simulink model "sha2_net_design"  (R2018b)
settings: Solver=VariableStepAuto  StartTime=0.0  StopTime=10.0  RelTol=1e-3
settings Model: Creator=Mihail  LastModifiedBy=Mihail

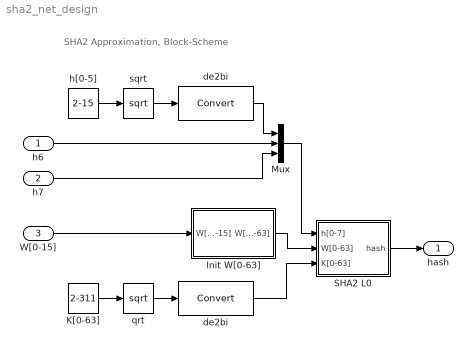
== system sha2_net_design ==
  note: SHA2 Approximation, Block-Scheme
  h6 : Inport
  h7 : Inport  Port=2
  W[0-15] : Inport  Port=3
  Init W[0-63] : Subsystem
  K[0-63] : Constant  Value=2-311
  Mux : Mux  Inputs=3
  SHA2 L0 : Subsystem
  de2bi : DataTypeConversion
  "de2bi " : DataTypeConversion
  h[0-5] : Constant  Value=2-15
  qrt : Sqrt  SaturateOnIntegerOverflow=on
  sqrt : Sqrt  SaturateOnIntegerOverflow=on
  hash : Outport
  wires:
  h[0-5]/1 -> sqrt/1
  K[0-63]/1 -> qrt/1
  sqrt/1 -> de2bi/1
  de2bi/1 -> Mux/1
  h6/1 -> Mux/2
  h7/1 -> Mux/3
  qrt/1 -> "de2bi "/1
  Init W[0-63]/1("W[0-63] ") -> SHA2 L0/2(W[0-63])
  Mux/1 -> SHA2 L0/1(h[0-7])
  "de2bi "/1 -> SHA2 L0/3(K[0-63])
  W[0-15]/1 -> Init W[0-63]/1(W[0-15])
  SHA2 L0/1(hash) -> hash/1

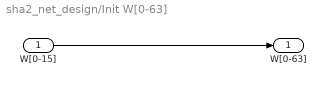
== system sha2_net_design/Init W[0-63] ==
  W[0-15] : Inport
  "W[0-63] " : Outport
  wires:
  W[0-15]/1 -> "W[0-63] "/1

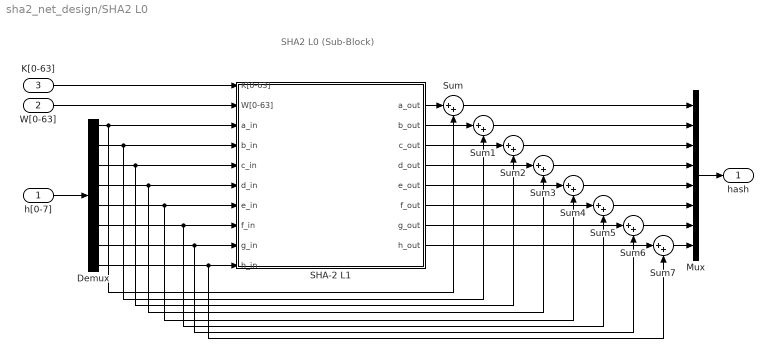
== system sha2_net_design/SHA2 L0 ==
  note: SHA2 L0 (Sub-Block)
  h[0-7] : Inport
  W[0-63] : Inport  Port=2
  K[0-63] : Inport  Port=3
  Demux : Demux  Outputs=8
  Mux : Mux  Inputs=8
  SHA-2 L1 : Subsystem
  Sum{,1..7} (8 alike) : Sum  Inputs=|++
  hash : Outport
  wires:
  SHA-2 L1/1(a_out) -> Sum/1
  SHA-2 L1/2(b_out) -> Sum1/1
  Sum/1 -> Mux/1
  Sum1/1 -> Mux/2
  Sum2/1 -> Mux/3
  SHA-2 L1/3(c_out) -> Sum2/1
  SHA-2 L1/4(d_out) -> Sum3/1
  Sum3/1 -> Mux/4
  SHA-2 L1/5(e_out) -> Sum4/1
  Sum4/1 -> Mux/5
  Mux/1 -> hash/1
  SHA-2 L1/6(f_out) -> Sum5/1
  Sum6/1 -> Mux/7
  Sum5/1 -> Mux/6
  Sum7/1 -> Mux/8
  SHA-2 L1/7(g_out) -> Sum6/1
  SHA-2 L1/8(h_out) -> Sum7/1
  W[0-63]/1 -> SHA-2 L1/2(W[0-63])
  K[0-63]/1 -> SHA-2 L1/1(K[0-63])
  h[0-7]/1 -> Demux/1
  Demux/1 -> Sum/2, SHA-2 L1/3(a_in)
  Demux/2 -> Sum1/2, SHA-2 L1/4(b_in)
  Demux/3 -> Sum2/2, SHA-2 L1/5(c_in)
  Demux/4 -> Sum3/2, SHA-2 L1/6(d_in)
  Demux/5 -> Sum4/2, SHA-2 L1/7(e_in)
  Demux/6 -> Sum5/2, SHA-2 L1/8(f_in)
  Demux/7 -> Sum6/2, SHA-2 L1/9(g_in)
  Demux/8 -> Sum7/2, SHA-2 L1/10(h_in)

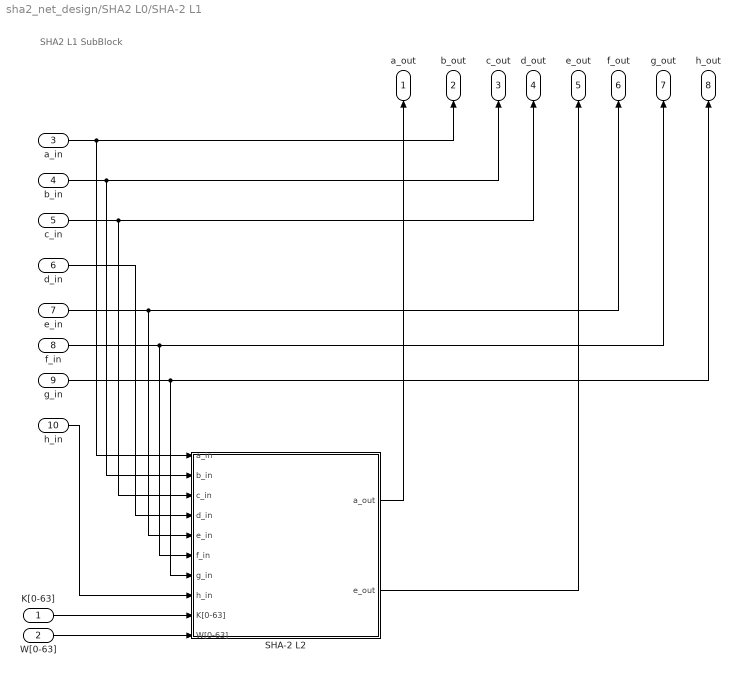
== system sha2_net_design/SHA2 L0/SHA-2 L1 ==
  note: SHA2 L1 SubBlock
  K[0-63] : Inport
  W[0-63] : Inport  Port=2
  a_in : Inport  Port=3
  b_in : Inport  Port=4
  c_in : Inport  Port=5
  d_in : Inport  Port=6
  e_in : Inport  Port=7
  f_in : Inport  Port=8
  g_in : Inport  Port=9
  h_in : Inport  Port=10
  SHA-2 L2 : Subsystem
  a_out : Outport
  b_out : Outport  Port=2
  c_out : Outport  Port=3
  d_out : Outport  Port=4
  e_out : Outport  Port=5
  f_out : Outport  Port=6
  g_out : Outport  Port=7
  h_out : Outport  Port=8
  wires:
  g_in/1 -> SHA-2 L2/7(g_in), h_out/1
  f_in/1 -> SHA-2 L2/6(f_in), g_out/1
  e_in/1 -> SHA-2 L2/5(e_in), f_out/1
  c_in/1 -> SHA-2 L2/3(c_in), d_out/1
  b_in/1 -> SHA-2 L2/2(b_in), c_out/1
  a_in/1 -> SHA-2 L2/1(a_in), b_out/1
  SHA-2 L2/1(a_out) -> a_out/1
  SHA-2 L2/2(e_out) -> e_out/1
  d_in/1 -> SHA-2 L2/4(d_in)
  h_in/1 -> SHA-2 L2/8(h_in)
  K[0-63]/1 -> SHA-2 L2/9(K[0-63])
  W[0-63]/1 -> SHA-2 L2/10(W[0-63])

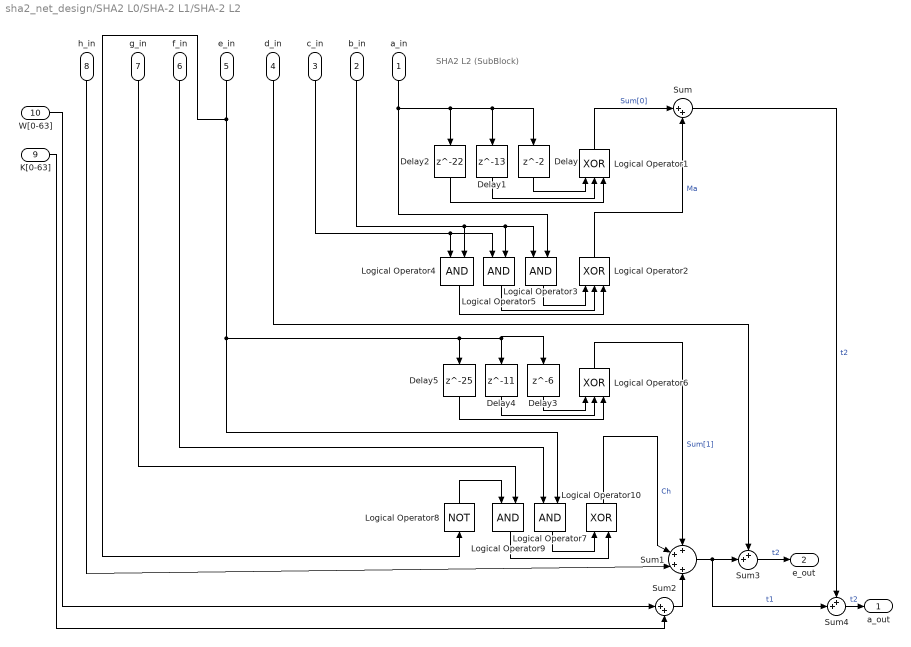
== system sha2_net_design/SHA2 L0/SHA-2 L1/SHA-2 L2 ==
  note: SHA2 L2 (SubBlock)
  a_in : Inport
  b_in : Inport  Port=2
  c_in : Inport  Port=3
  d_in : Inport  Port=4
  e_in : Inport  Port=5
  f_in : Inport  Port=6
  g_in : Inport  Port=7
  h_in : Inport  Port=8
  K[0-63] : Inport  Port=9
  W[0-63] : Inport  Port=10
  Delay : Delay
  Delay1 : Delay  DelayLength=13
  Delay2 : Delay  DelayLength=22
  Delay3 : Delay  DelayLength=6
  Delay4 : Delay  DelayLength=11
  Delay5 : Delay  DelayLength=25
  Logical Operator1 : Logic  Operator=XOR  Inputs=3  AllPortsSameDT=off  OutDataTypeStr=boolean
  Logical Operator10 : Logic  Operator=XOR  AllPortsSameDT=off  OutDataTypeStr=boolean
  Logical Operator2 : Logic  Operator=XOR  Inputs=3  AllPortsSameDT=off  OutDataTypeStr=boolean
  Logical Operator{3..5,7,9} (5 alike) : Logic  AllPortsSameDT=off  OutDataTypeStr=boolean
  Logical Operator6 : Logic  Operator=XOR  Inputs=3  AllPortsSameDT=off  OutDataTypeStr=boolean
  Logical Operator8 : Logic  Operator=NOT  Inputs=3  AllPortsSameDT=off  OutDataTypeStr=boolean
  Sum : Sum  Inputs=|++
  Sum1 : Sum  Inputs=++++
  Sum2 : Sum  Inputs=|++
  Sum3 : Sum  Inputs=++|
  Sum4 : Sum  Inputs=++|
  a_out : Outport
  e_out : Outport  Port=2
  wires:
  a_in/1 -> Logical Operator3/2, Delay/1, Delay1/1, Delay2/1
  Delay/1 -> Logical Operator1/1
  Delay1/1 -> Logical Operator1/2
  Delay2/1 -> Logical Operator1/3
  b_in/1 -> Logical Operator5/2, Logical Operator3/1, Logical Operator4/2
  c_in/1 -> Logical Operator5/1, Logical Operator4/1
  Logical Operator3/1 -> Logical Operator2/1
  Logical Operator5/1 -> Logical Operator2/2
  Logical Operator4/1 -> Logical Operator2/3
  e_in/1 -> Logical Operator8/1, Logical Operator7/2, Delay3/1, Delay4/1, Delay5/1
  Delay3/1 -> Logical Operator6/1
  Delay4/1 -> Logical Operator6/2
  Delay5/1 -> Logical Operator6/3
  f_in/1 -> Logical Operator7/1
  g_in/1 -> Logical Operator9/2
  Logical Operator8/1 -> Logical Operator9/1
  Logical Operator7/1 -> Logical Operator10/1
  Logical Operator9/1 -> Logical Operator10/2
  Logical Operator1/1 -> Sum/1  "Sum[0]"
  Logical Operator2/1 -> Sum/2  "Ma"
  Sum/1 -> Sum4/1  "t2"
  W[0-63]/1 -> Sum2/1
  K[0-63]/1 -> Sum2/2
  Sum2/1 -> Sum1/4
  Logical Operator6/1 -> Sum1/1  "Sum[1]"
  Logical Operator10/1 -> Sum1/2  "Ch"
  h_in/1 -> Sum1/3
  Sum3/1 -> e_out/1  "t2"
  Sum4/1 -> a_out/1  "t2"
  Sum1/1 -> Sum4/2, Sum3/2  "t1"
  d_in/1 -> Sum3/1
